simulink model "final_test"  (R2017a)
settings: Solver=VariableStepAuto  StartTime=0.0  StopTime=10.0  RelTol=1e-3
settings Model: Creator=ashwi  LastModifiedBy=ashwi

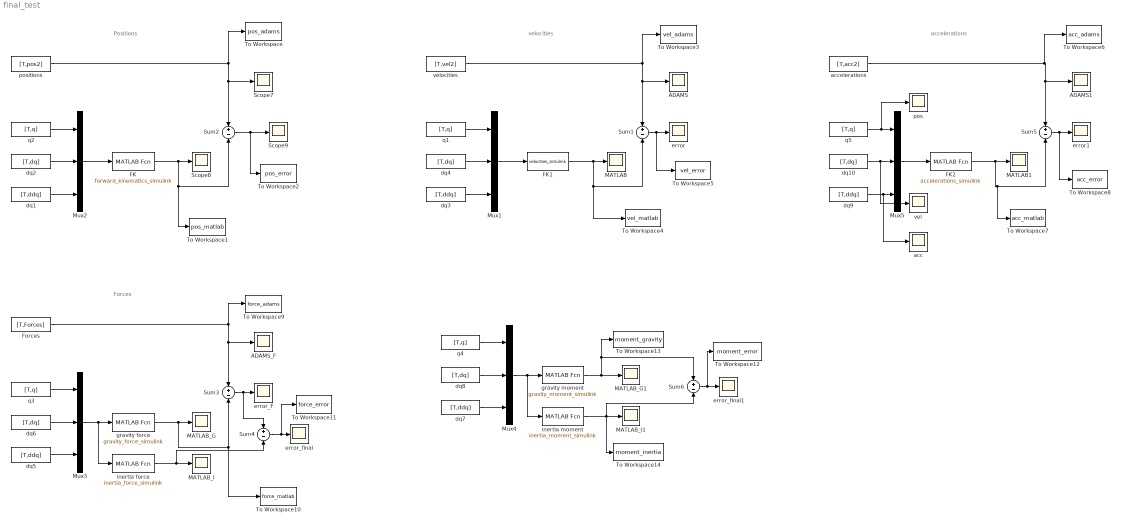
== system final_test ==
  note: Positions
  note: velocities
  note: Forces
  note: accelerations
  ADAMS : Scope
  ADAMS1 : Scope
  ADAMS_F : Scope
  FK : MATLABFcn  MATLABFcn=forward_kinematics_simulink
  FK1 : MATLABFcn  MATLABFcn=velocities_simulink
  FK2 : MATLABFcn  MATLABFcn=accelerations_simulink
  Forces : FromWorkspace  VariableName=[T,Forces]  SampleTime=0
  MATLAB : Scope
  MATLAB1 : Scope
  MATLAB_G : Scope
  MATLAB_G1 : Scope
  MATLAB_I : Scope
  MATLAB_I1 : Scope
  Mux{1..5} (5 alike) : Mux  Inputs=3
  Scope7 : Scope
  Scope8 : Scope
  Scope9 : Scope
  Sum{1..6} (6 alike) : Sum  Inputs=+-
  To Workspace : ToWorkspace  VariableName=pos_adams  SaveFormat=Timeseries  SampleTime=-1
  To Workspace1 : ToWorkspace  VariableName=pos_matlab  SaveFormat=Timeseries  SampleTime=-1
  To Workspace10 : ToWorkspace  VariableName=force_matlab  SaveFormat=Timeseries  SampleTime=-1
  To Workspace11 : ToWorkspace  VariableName=force_error  SaveFormat=Timeseries  SampleTime=-1
  To Workspace12 : ToWorkspace  VariableName=moment_error  SaveFormat=Timeseries  SampleTime=-1
  To Workspace13 : ToWorkspace  VariableName=moment_gravity  SaveFormat=Timeseries  SampleTime=-1
  To Workspace14 : ToWorkspace  VariableName=moment_inertia  SaveFormat=Timeseries  SampleTime=-1
  To Workspace2 : ToWorkspace  VariableName=pos_error  SaveFormat=Timeseries  SampleTime=-1
  To Workspace3 : ToWorkspace  VariableName=vel_adams  SaveFormat=Timeseries  SampleTime=-1
  To Workspace4 : ToWorkspace  VariableName=vel_matlab  SaveFormat=Timeseries  SampleTime=-1
  To Workspace5 : ToWorkspace  VariableName=vel_error  SaveFormat=Timeseries  SampleTime=-1
  To Workspace6 : ToWorkspace  VariableName=acc_adams  SaveFormat=Timeseries  SampleTime=-1
  To Workspace7 : ToWorkspace  VariableName=acc_matlab  SaveFormat=Timeseries  SampleTime=-1
  To Workspace8 : ToWorkspace  VariableName=acc_error  SaveFormat=Timeseries  SampleTime=-1
  To Workspace9 : ToWorkspace  VariableName=force_adams  SaveFormat=Timeseries  SampleTime=-1
  acc : Scope
  accelerations : FromWorkspace  VariableName=[T,acc2]  SampleTime=0
  dq{1,3,5,7,9} (5 alike) : FromWorkspace  VariableName=[T,ddq]  SampleTime=0
  dq{2,4,6,8,10} (5 alike) : FromWorkspace  VariableName=[T,dq]  SampleTime=0
  error : Scope
  error1 : Scope
  error_F : Scope
  error_final : Scope
  error_final1 : Scope
  gravity force : MATLABFcn  MATLABFcn=gravity_force_simulink
  gravity moment : MATLABFcn  MATLABFcn=gravity_moment_simulink
  inertia force : MATLABFcn  MATLABFcn=inertia_force_simulink
  inertia moment : MATLABFcn  MATLABFcn=inertia_moment_simulink
  pos : Scope
  positions : FromWorkspace  VariableName=[T,pos2]  SampleTime=0
  q{1..5} (5 alike) : FromWorkspace  VariableName=[T,q]  SampleTime=0
  vel : Scope
  velocities : FromWorkspace  VariableName=[T,vel2]  SampleTime=0
  wires:
  q2/1 -> Mux2/1
  positions/1 -> To Workspace/1, Sum2/1, Scope7/1
  Sum2/1 -> To Workspace2/1, Scope9/1
  dq2/1 -> Mux2/2
  dq1/1 -> Mux2/3
  Mux2/1 -> FK/1
  FK/1 -> To Workspace1/1, Sum2/2, Scope8/1
  velocities/1 -> To Workspace3/1, Sum1/1, ADAMS/1
  FK1/1 -> To Workspace4/1, Sum1/2, MATLAB/1
  Mux1/1 -> FK1/1
  q1/1 -> Mux1/1
  dq4/1 -> Mux1/2
  Sum1/1 -> To Workspace5/1, error/1
  dq3/1 -> Mux1/3
  gravity force/1 -> To Workspace10/1, Sum3/2, MATLAB_G/1
  Mux3/1 -> inertia force/1, gravity force/1
  q3/1 -> Mux3/1
  dq6/1 -> Mux3/2
  Sum3/1 -> Sum4/1, error_F/1
  dq5/1 -> Mux3/3
  inertia force/1 -> Sum4/2, MATLAB_I/1
  Sum4/1 -> To Workspace11/1, error_final/1
  dq7/1 -> Mux4/3
  gravity moment/1 -> To Workspace13/1, Sum6/1, MATLAB_G1/1
  q4/1 -> Mux4/1
  Mux4/1 -> inertia moment/1, gravity moment/1
  Sum6/1 -> To Workspace12/1, error_final1/1
  q5/1 -> pos/1, Mux5/1
  accelerations/1 -> To Workspace6/1, Sum5/1, ADAMS1/1
  Sum5/1 -> To Workspace8/1, error1/1
  Mux5/1 -> FK2/1
  FK2/1 -> To Workspace7/1, Sum5/2, MATLAB1/1
  dq10/1 -> vel/1, Mux5/2
  dq9/1 -> acc/1, Mux5/3
  dq8/1 -> Mux4/2
  Forces/1 -> To Workspace9/1, Sum3/1, ADAMS_F/1
  inertia moment/1 -> To Workspace14/1, Sum6/2, MATLAB_I1/1
